simulink model "Copy_of_Ball_Estimation_27_12_new"  (Simulink 8.0)
settings: Solver=ode4  StartTime=0.0  StopTime=inf  FixedStep=sample_time  RelTol=1e-3
InitFcn:
  | sample_time=0.005;%0.004;%0.0025;%0.02;
  | sample_time_Vicon = 0.005;
  | DeltaT = 0.02;
  | g = 9.81;
  | H0 = g%0.3165;
  | 
  | Q6_mass = 0.7;
  | 
  | Q6_Omega_r = 1.6; %for horizon ref
  | Q6_Zeta_r = 0.5; %for horizon ref
  | Q6_Omega_r_h = 2;%for vertical ref
  | Q6_Zeta_r_h = 1; %for vertical ref
  | 
  | 
  | Q6_Omega = 1.5; %for horizon control
  | Q6_Zeta = 0.5; %for horizon control
  | Q6_Omega_h= 2; %for vertical control
  | Q6_Zeta_h = 0.7; %for vertical control
  | 
  | 
  | Q6_acc_max = 5;%horizontal max acc
  | Q6_acc_max_h = 3;%horizontal max acc
  | 
  | omega_circle = 72*pi/180;
  | omega_h = 0.1;%Ascending speed
  | PI = pi;
  | Circle_R = 2.5;
  | MAX_Height = -2;
libraries: simulink x2, dspadpt3 x2
settings Model: Creator=ttcl3  LastModifiedBy=NTU User
settings SolverCC: MaxConsecutiveMinStep=auto
settings DataIOCC: SignalLoggingSaveFormat=ModelDataLogs
settings DebuggingCC: MultiTaskRateTransMsg=warning  FcnCallInpInsideContextMsg=UseLocalSettings
settings SFSimCC: SimParseCustomCode=off
settings CodeAppCC: CustomSymbolStrType=$N$R$M_T  InternalIdentifier=Shortened
settings GRTTargetCC: CombineOutputUpdateFcns=off  GRTInterface=on

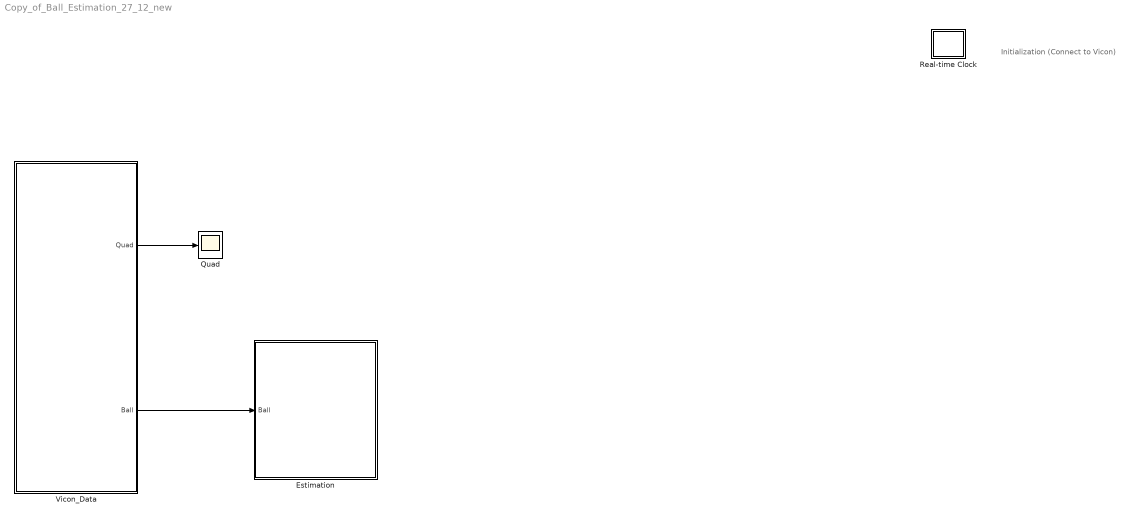
== system Copy_of_Ball_Estimation_27_12_new ==
  note: Initialization
      | (Connect to Vicon)
  Estimation : Subsystem
  Quad : Scope
      settings: YMin=0  YMax=3.25  MaxDataPoints=50000
  Real-time Clock : Subsystem  mask(Real-time Clock){sample_time=0.02, tolerance=1}
      mask prompts: sample_time "Synchronize with real-time every n seconds:"; tolerance "Real-time warning tolerance (seconds):"
      mask help: Real-time Synchronization Block
      mask Help: This block synchronizes simulation time with the PC real-time clock or UNIX system clock. The first dialog entry is the period at which the clock is checked to insure real-time synchronization. The second dialog entry is the number of seconds that the simulation time must be within real-time before a warning is printed.
      mask Display: plot(0,0,100,100,[40,60,60,54,54,64,69,76,82,77,81,83,83,81,78,74,70,64,57,49,41,35,32,30,30,31,34,40,47,47,40,40],[90,90,85,85,80,79,76,87,80,70,64,57,49,41,33,28,24,22,21,23,25,31,37,46,56,65,73,78,80,85,85,90],[69,53,53],[64,50,73])
  Vicon_Data : Subsystem
  wires:
  Vicon_Data/2(Ball) -> Estimation/1(Ball)
  Vicon_Data/1(Quad) -> Quad/1

== system Copy_of_Ball_Estimation_27_12_new/Estimation ==
  Ball : Inport
  Bus Selector1 : BusSelector  OutputSignals=Position,Velocity
  Trajectory Logic1 : Subsystem
  wires:
  Ball/1 -> Bus Selector1/1
  Bus Selector1/1 -> Trajectory Logic1/1(Ball_Pos)  "<Position>"
  Bus Selector1/2 -> Trajectory Logic1/2(Ball_Vel)  "<Velocity>"

== system Copy_of_Ball_Estimation_27_12_new/Real-time Clock ==
  Real-time Clock : S-Function  FunctionName=rtclock  Parameters=sample_time, tolerance  EnableBusSupport=off

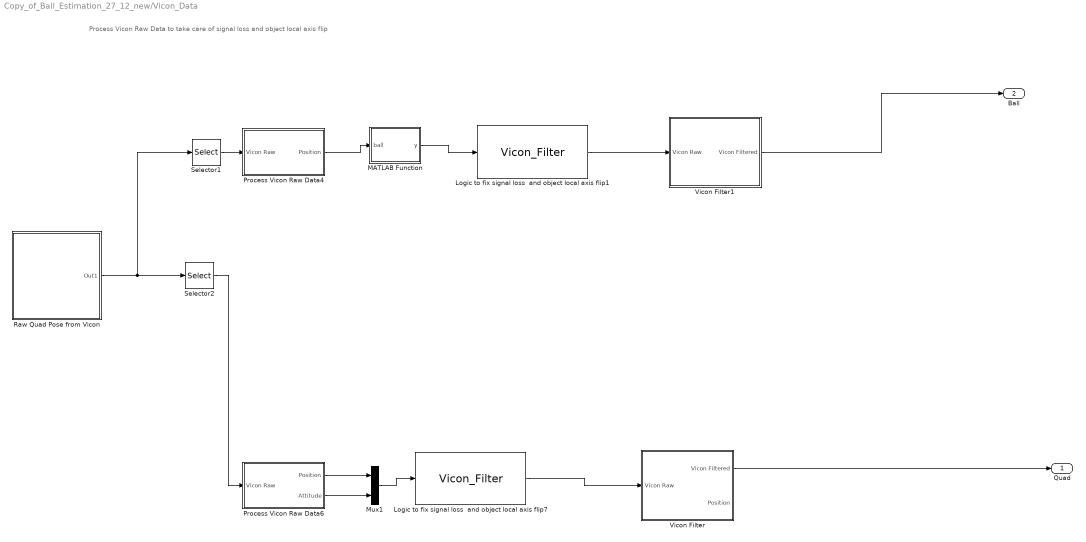
== system Copy_of_Ball_Estimation_27_12_new/Vicon_Data ==
  note: Process Vicon Raw Data to take care of signal loss and object local axis flip
  Logic to fix signal loss  and object local axis flip1 : M-S-Function  FunctionName=Vicon_Filter
  Logic to fix signal loss  and object local axis flip7 : M-S-Function  FunctionName=Vicon_Filter
  MATLAB Function : MATLAB Function  TreatAsAtomicUnit=on
  Mux1 : Mux  Inputs=2
  Process Vicon Raw Data4 : Subsystem
  Process Vicon Raw Data6 : Subsystem
  Raw Quad Pose from Vicon : Subsystem
  Selector1 : Selector  InputPortWidth=9  IndexOptions=Index vector (dialog)  Indices=[7 8 9]  OutputSizes=1
  Selector2 : Selector  InputPortWidth=9  IndexOptions=Index vector (dialog)  Indices=[1 2 3 4 5 6]  OutputSizes=1
  Vicon Filter : Subsystem  AncestorBlock=X330_Control/Vicon Filter
  Vicon Filter1 : Subsystem  AncestorBlock=X330_Control/Vicon Filter
  Quad : Outport
  Ball : Outport  Port=2
  wires:
  Selector2/1 -> Process Vicon Raw Data6/1(Vicon Raw)
  Logic to fix signal loss  and object local axis flip7/1 -> Vicon Filter/1(Vicon Raw)
  Process Vicon Raw Data6/1(Position) -> Mux1/1
  Process Vicon Raw Data6/2(Attitude) -> Mux1/2
  Mux1/1 -> Logic to fix signal loss  and object local axis flip7/1
  Vicon Filter/1(Vicon Filtered) -> Quad/1
  Process Vicon Raw Data4/1(Position) -> MATLAB Function/1(ball)
  Vicon Filter1/1(Vicon Filtered) -> Ball/1
  Raw Quad Pose from Vicon/1(Out1) -> Selector1/1, Selector2/1
  Selector1/1 -> Process Vicon Raw Data4/1(Vicon Raw)
  MATLAB Function/1(y) -> Logic to fix signal loss  and object local axis flip1/1
  Logic to fix signal loss  and object local axis flip1/1 -> Vicon Filter1/1(Vicon Raw)

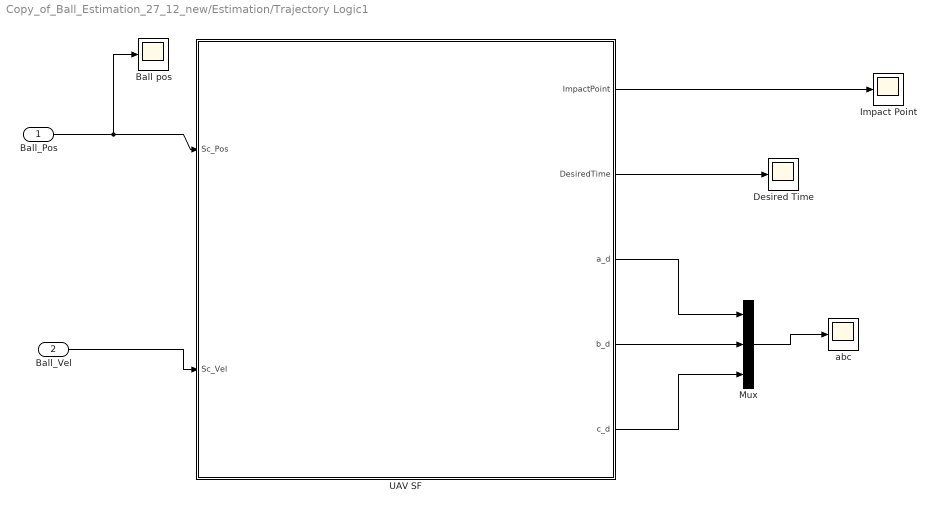
== system Copy_of_Ball_Estimation_27_12_new/Estimation/Trajectory Logic1 ==
  Ball_Pos : Inport
  Ball_Vel : Inport  Port=2
  Ball pos : Scope
      settings: TimeRange=10  YMin=-4.5  SaveName=ScopeData4  MaxDataPoints=50000
  Desired Time : Scope
      settings: TimeRange=14.55830388692581  YMin=-0.05018891687657431  YMax=0.1552267002518891  SaveName=ScopeData5  MaxDataPoints=50000
  Impact Point : Scope
      settings: TimeRange=1.719691973284533  YMin=-3.5  YMax=3.5  SaveName=ScopeData2  MaxDataPoints=50000
  Mux : Mux  Inputs=3
  UAV SF : Stateflow chart  TreatAsAtomicUnit=on
  abc : Scope
      settings: YMin=-0.25  YMax=4.5  MaxDataPoints=50000
  wires:
  Ball_Pos/1 -> Ball pos/1, UAV SF/1(Sc_Pos)
  Ball_Vel/1 -> UAV SF/2(Sc_Vel)
  UAV SF/2(DesiredTime) -> Desired Time/1
  UAV SF/3(a_d) -> Mux/1
  UAV SF/4(b_d) -> Mux/2
  UAV SF/5(c_d) -> Mux/3
  Mux/1 -> abc/1
  UAV SF/1(ImpactPoint) -> Impact Point/1

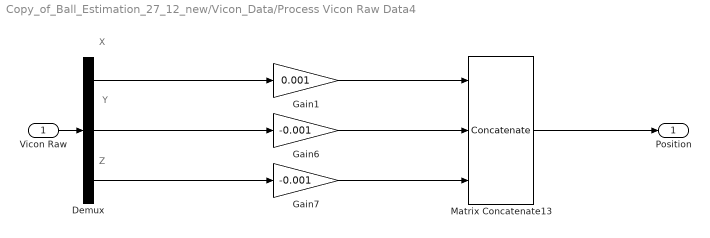
== system Copy_of_Ball_Estimation_27_12_new/Vicon_Data/Process Vicon Raw Data4 ==
  note: X
  note: Y
  note: Z
  Vicon Raw : Inport
  Demux : Demux  Outputs=3
  Gain1 : Gain  Gain=0.001
  Gain6 : Gain  Gain=-0.001
  Gain7 : Gain  Gain=-0.001
  Matrix Concatenate13 : Concatenate  NumInputs=3  Mode=Multidimensional array
  Position : Outport
  wires:
  Gain1/1 -> Matrix Concatenate13/1
  Demux/1 -> Gain1/1
  Demux/2 -> Gain6/1
  Demux/3 -> Gain7/1
  Gain6/1 -> Matrix Concatenate13/2
  Gain7/1 -> Matrix Concatenate13/3
  Matrix Concatenate13/1 -> Position/1
  Vicon Raw/1 -> Demux/1

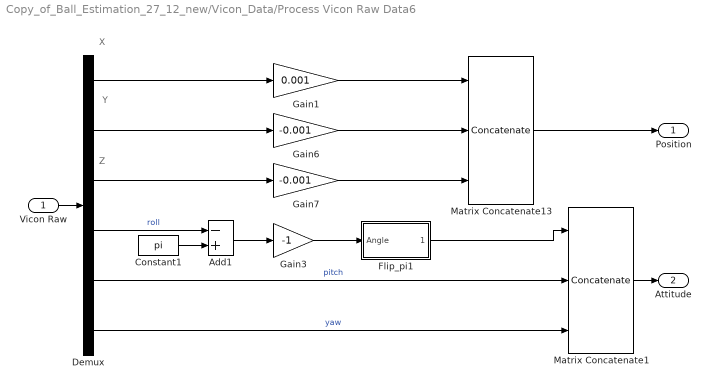
== system Copy_of_Ball_Estimation_27_12_new/Vicon_Data/Process Vicon Raw Data6 ==
  note: X
  note: Y
  note: Z
  Vicon Raw : Inport
  Add1 : Sum  Inputs=-+
  Constant1 : Constant  Value=pi  OutDataTypeStr=double
  Demux : Demux  Outputs=6
  Flip_pi1 : Subsystem  mask(Flip -pi to pi){}
      mask help: Flips the inputs into the range -pi to pi
      mask Help: Flips the inputs into the range -pi to pi
      mask Display: disp('Flip_pi')
  Gain1 : Gain  Gain=0.001
  Gain3 : Gain  Gain=-1
  Gain6 : Gain  Gain=-0.001
  Gain7 : Gain  Gain=-0.001
  Matrix Concatenate1 : Concatenate  NumInputs=3  Mode=Multidimensional array
  Matrix Concatenate13 : Concatenate  NumInputs=3  Mode=Multidimensional array
  Position : Outport
  Attitude : Outport  Port=2
  wires:
  Constant1/1 -> Add1/2
  Demux/6 -> Matrix Concatenate1/3  "yaw"
  Gain1/1 -> Matrix Concatenate13/1
  Demux/1 -> Gain1/1
  Demux/2 -> Gain6/1
  Demux/3 -> Gain7/1
  Demux/4 -> Add1/1  "roll"
  Gain6/1 -> Matrix Concatenate13/2
  Gain7/1 -> Matrix Concatenate13/3
  Add1/1 -> Gain3/1
  Gain3/1 -> Flip_pi1/1(Angle)
  Demux/5 -> Matrix Concatenate1/2  "pitch"
  Flip_pi1/1(Angle_Flip) -> Matrix Concatenate1/1
  Matrix Concatenate13/1 -> Position/1
  Vicon Raw/1 -> Demux/1
  Matrix Concatenate1/1 -> Attitude/1

== system Copy_of_Ball_Estimation_27_12_new/Vicon_Data/Raw Quad Pose from Vicon ==
  Constant : Constant
  Interpreted MATLAB Function : MATLABFcn  MATLABFcn=GetViconPose_BallCatching_mae_lab  OutputDimensions=9  SampleTime=0.005
  Out1 : Outport
  wires:
  Constant/1 -> Interpreted MATLAB Function/1
  Interpreted MATLAB Function/1 -> Out1/1

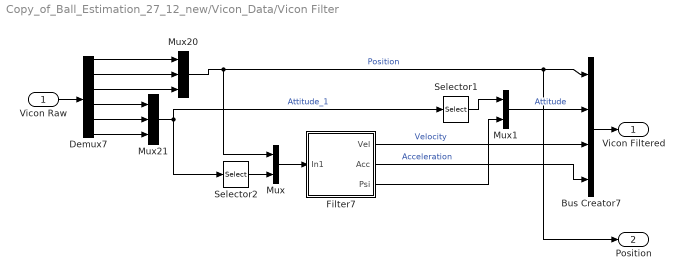
== system Copy_of_Ball_Estimation_27_12_new/Vicon_Data/Vicon Filter ==
  Vicon Raw : Inport
  Bus Creator7 : BusCreator
  Demux7 : Demux  Outputs=6
  Filter7 : Subsystem
  Mux : Mux  Inputs=2
  Mux1 : Mux  Inputs=2
  Mux20 : Mux  Inputs=3
  Mux21 : Mux  Inputs=3
  Selector1 : Selector  InputPortWidth=3  IndexOptions=Index vector (dialog)  Indices=[1 2]  OutputSizes=1
  Selector2 : Selector  InputPortWidth=3  IndexOptions=Index vector (dialog)  Indices=[3]  OutputSizes=1
  Vicon Filtered : Outport
  Position : Outport  Port=2
  wires:
  Bus Creator7/1 -> Vicon Filtered/1
  Vicon Raw/1 -> Demux7/1
  Mux1/1 -> Bus Creator7/2  "Attitude"
  Selector1/1 -> Mux1/1
  Filter7/3(Psi) -> Mux1/2
  Mux/1 -> Filter7/1(In1)
  Selector2/1 -> Mux/2
  Filter7/2(Acc) -> Bus Creator7/4  "Acceleration"
  Filter7/1(Vel) -> Bus Creator7/3  "Velocity"
  Mux21/1 -> Selector1/1, Selector2/1  "Attitude_1"
  Mux20/1 -> Mux/1, Position/1, Bus Creator7/1  "Position"
  Demux7/2 -> Mux20/2
  Demux7/1 -> Mux20/1
  Demux7/6 -> Mux21/3
  Demux7/5 -> Mux21/2
  Demux7/4 -> Mux21/1
  Demux7/3 -> Mux20/3

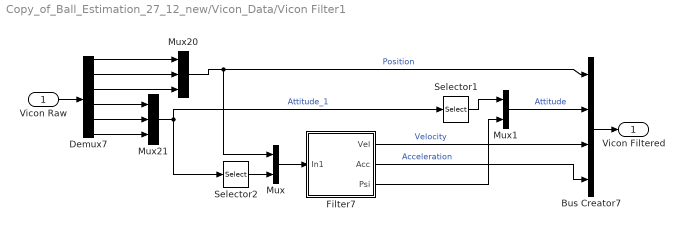
== system Copy_of_Ball_Estimation_27_12_new/Vicon_Data/Vicon Filter1 ==
  Vicon Raw : Inport
  Bus Creator7 : BusCreator
  Demux7 : Demux  Outputs=6
  Filter7 : Subsystem
  Mux : Mux  Inputs=2
  Mux1 : Mux  Inputs=2
  Mux20 : Mux  Inputs=3
  Mux21 : Mux  Inputs=3
  Selector1 : Selector  InputPortWidth=3  IndexOptions=Index vector (dialog)  Indices=[1 2]  OutputSizes=1
  Selector2 : Selector  InputPortWidth=3  IndexOptions=Index vector (dialog)  Indices=[3]  OutputSizes=1
  Vicon Filtered : Outport
  wires:
  Demux7/3 -> Mux20/3
  Demux7/4 -> Mux21/1
  Demux7/5 -> Mux21/2
  Demux7/6 -> Mux21/3
  Demux7/1 -> Mux20/1
  Demux7/2 -> Mux20/2
  Mux20/1 -> Bus Creator7/1, Mux/1  "Position"
  Mux21/1 -> Selector2/1, Selector1/1  "Attitude_1"
  Filter7/1(Vel) -> Bus Creator7/3  "Velocity"
  Filter7/2(Acc) -> Bus Creator7/4  "Acceleration"
  Selector2/1 -> Mux/2
  Mux/1 -> Filter7/1(In1)
  Filter7/3(Psi) -> Mux1/2
  Selector1/1 -> Mux1/1
  Mux1/1 -> Bus Creator7/2  "Attitude"
  Vicon Raw/1 -> Demux7/1
  Bus Creator7/1 -> Vicon Filtered/1

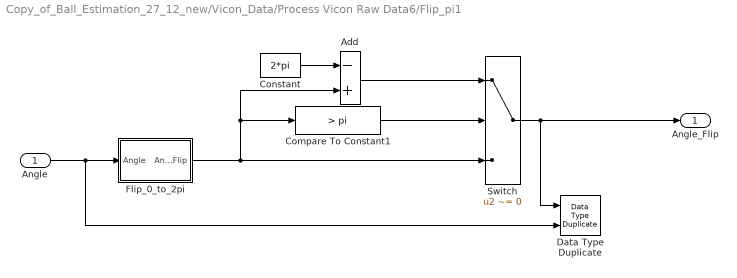
== system Copy_of_Ball_Estimation_27_12_new/Vicon_Data/Process Vicon Raw Data6/Flip_pi1 ==
  Angle : Inport
  Add : Sum  Inputs=-+
  Compare To Constant1 : simulink/Logic and Bit Operations/Compare To Constant  relop=>  const=pi  OutDataTypeStr=uint8  ZeroCross=off
  Constant : Constant  Value=2*pi
  Data Type Duplicate : DataTypeDuplicate
  Flip_0_to_2pi : Subsystem  mask(Flip zero to 2pi){}
      mask help: Flips the inputs into the range zero to +2pi
      mask Help: Flips the inputs into the range zero to +2pi
      mask Display: disp('Flip_0_2pi')
  Switch : Switch  Criteria=u2 ~= 0
  Angle_Flip : Outport
  wires:
  Switch/1 -> Data Type Duplicate/1, Angle_Flip/1
  Add/1 -> Switch/1
  Constant/1 -> Add/1
  Compare To Constant1/1 -> Switch/2
  Flip_0_to_2pi/1(Angle_Flip) -> Add/2, Compare To Constant1/1, Switch/3
  Angle/1 -> Data Type Duplicate/2, Flip_0_to_2pi/1(Angle)

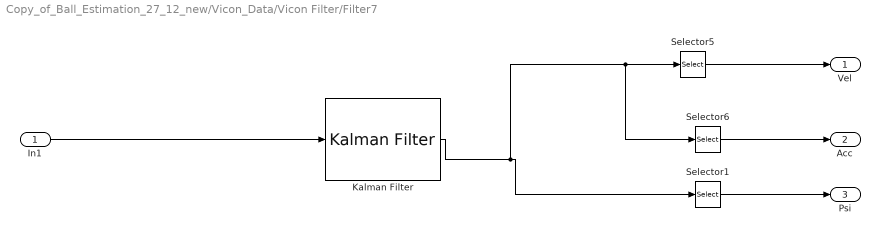
== system Copy_of_Ball_Estimation_27_12_new/Vicon_Data/Vicon Filter/Filter7 ==
  In1 : Inport
  Kalman Filter : dspadpt3/Kalman Filter  num_targets=1  sourceEnable=Always  isReset=on  X=zeros([12, 1])  P=zeros(12)  A=[1 sample_time_Vicon sample_time_Vicon*sample_time_Vicon/2 zeros(1,9);0 1 sample_time_Vicon zeros(1,9);0 0 1 zeros(1,9);0 0 0 1 sample_time_Vicon sample_time_Vicon*sample_time_Vicon/2 zeros(1,6);zeros(1,4) 1 sample_time_Vicon zeros(1,6);zeros(1,5) 1 zeros(1,6);zeros(1,6) 1 sample_time_Vicon sample_time_Vicon*sample_time_Vicon/2 zeros(1,3);zeros(1,7) 1 sample_time_Vicon zeros(1,3);zeros(1,8) 1 zeros(1,3);zeros(1,9) 1 sample_time_Vicon sample_time_Vicon*sample_time_Vicon/2;zeros(1,10) 1 sample_time_Vicon;zeros(1,11) 1];  sourceMeasure=Specify via Dialog  H=[1 zeros(1,11); zeros(1,3) 1 zeros(1,8);zeros(1,6) 1 zeros(1,5);zeros(1,9) 1 0 0]  Q=diag([0 0.001 0.001 0 0.001 0.001 0 0.001 0.001 0 0.001 0.001]);  R=diag([0.001 0.001 0.001 0.05])  isOutputEstMeasure=off  isOutputEstState=on  isOutputEstError=off  isOutputPrdMeasure=off  isOutputPrdState=off  isOutputPrdError=off
  Selector1 : Selector  InputPortWidth=12  IndexOptions=Index vector (dialog)  Indices=[10]  OutputSizes=1
  Selector5 : Selector  InputPortWidth=12  IndexOptions=Index vector (dialog)  Indices=[2 5 8]  OutputSizes=1
  Selector6 : Selector  InputPortWidth=12  IndexOptions=Index vector (dialog)  Indices=[3 6 9]  OutputSizes=1
  Vel : Outport
  Acc : Outport  Port=2
  Psi : Outport  Port=3
  wires:
  Selector1/1 -> Psi/1
  Selector5/1 -> Vel/1
  In1/1 -> Kalman Filter/1
  Kalman Filter/1 -> Selector1/1, Selector5/1, Selector6/1
  Selector6/1 -> Acc/1

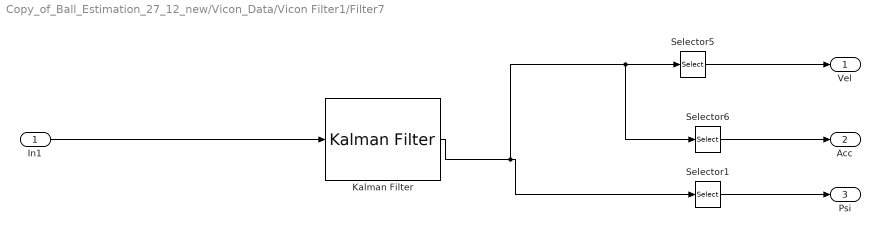
== system Copy_of_Ball_Estimation_27_12_new/Vicon_Data/Vicon Filter1/Filter7 ==
  In1 : Inport
  Kalman Filter : dspadpt3/Kalman Filter  num_targets=1  sourceEnable=Always  isReset=on  X=zeros([12, 1])  P=zeros(12)  A=[1 sample_time_Vicon sample_time_Vicon*sample_time_Vicon/2 zeros(1,9);0 1 sample_time_Vicon zeros(1,9);0 0 1 zeros(1,9);0 0 0 1 sample_time_Vicon sample_time_Vicon*sample_time_Vicon/2 zeros(1,6);zeros(1,4) 1 sample_time_Vicon zeros(1,6);zeros(1,5) 1 zeros(1,6);zeros(1,6) 1 sample_time_Vicon sample_time_Vicon*sample_time_Vicon/2 zeros(1,3);zeros(1,7) 1 sample_time_Vicon zeros(1,3);zeros(1,8) 1 zeros(1,3);zeros(1,9) 1 sample_time_Vicon sample_time_Vicon*sample_time_Vicon/2;zeros(1,10) 1 sample_time_Vicon;zeros(1,11) 1];  sourceMeasure=Specify via Dialog  H=[1 zeros(1,11); zeros(1,3) 1 zeros(1,8);zeros(1,6) 1 zeros(1,5);zeros(1,9) 1 0 0]  Q=diag([0 0.001 0.001 0 0.001 0.001 0 0.001 0.001 0 0.001 0.001]);  R=diag([0.001 0.001 0.001 0.05])  isOutputEstMeasure=off  isOutputEstState=on  isOutputEstError=off  isOutputPrdMeasure=off  isOutputPrdState=off  isOutputPrdError=off
  Selector1 : Selector  InputPortWidth=12  IndexOptions=Index vector (dialog)  Indices=[10]  OutputSizes=1
  Selector5 : Selector  InputPortWidth=12  IndexOptions=Index vector (dialog)  Indices=[2 5 8]  OutputSizes=1
  Selector6 : Selector  InputPortWidth=12  IndexOptions=Index vector (dialog)  Indices=[3 6 9]  OutputSizes=1
  Vel : Outport
  Acc : Outport  Port=2
  Psi : Outport  Port=3
  wires:
  Selector6/1 -> Acc/1
  Kalman Filter/1 -> Selector6/1, Selector5/1, Selector1/1
  In1/1 -> Kalman Filter/1
  Selector5/1 -> Vel/1
  Selector1/1 -> Psi/1

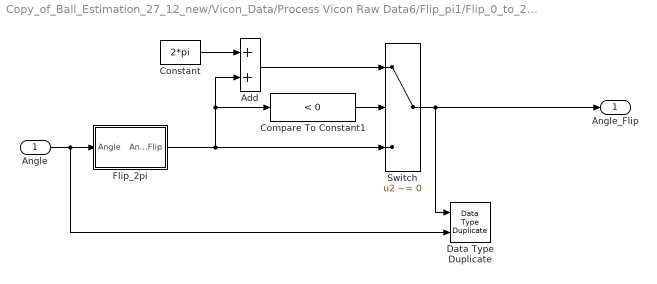
== system Copy_of_Ball_Estimation_27_12_new/Vicon_Data/Process Vicon Raw Data6/Flip_pi1/Flip_0_to_2pi ==
  Angle : Inport
  Add : Sum
  Compare To Constant1 : simulink/Logic and Bit Operations/Compare To Constant  relop=<  const=0  OutDataTypeStr=uint8  ZeroCross=off
  Constant : Constant  Value=2*pi
  Data Type Duplicate : DataTypeDuplicate
  Flip_2pi : Subsystem  mask(Flip -2pi to 2pi){}
      mask help: Flips the inputs into the range -2pi to +2pi
      mask Help: Flips the inputs into the range -2pi to +2pi
      mask Display: disp('Flip_2pi')
  Switch : Switch  Criteria=u2 ~= 0
  Angle_Flip : Outport
  wires:
  Switch/1 -> Data Type Duplicate/1, Angle_Flip/1
  Angle/1 -> Data Type Duplicate/2, Flip_2pi/1(Angle)
  Add/1 -> Switch/1
  Constant/1 -> Add/1
  Compare To Constant1/1 -> Switch/2
  Flip_2pi/1(Angle_Flip) -> Switch/3, Add/2, Compare To Constant1/1

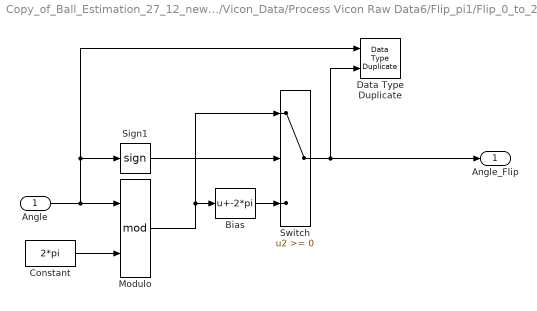
== system Copy_of_Ball_Estimation_27_12_new/Vicon_Data/Process Vicon Raw Data6/Flip_pi1/Flip_0_to_2pi/Flip_2pi ==
  Angle : Inport
  Bias : Bias  Bias=-2*pi
  Constant : Constant  Value=2*pi
  Data Type Duplicate : DataTypeDuplicate
  Modulo : Math  Operator=mod  SaturateOnIntegerOverflow=on
  Sign1 : Signum
  Switch : Switch
  Angle_Flip : Outport
  wires:
  Switch/1 -> Data Type Duplicate/2, Angle_Flip/1
  Bias/1 -> Switch/3
  Sign1/1 -> Switch/2
  Modulo/1 -> Switch/1, Bias/1
  Constant/1 -> Modulo/2
  Angle/1 -> Data Type Duplicate/1, Sign1/1, Modulo/1

== matlab function Vicon_Data/MATLAB Function ==
  data: ball input double; y output double
function y = fcn(ball)
%#codegen
temp = zeros(3,1);

for i=1:3;
   temp(i) = ball(i);     
end;
y = zeros(6,1);
y(1) = temp(1);
y(2) = temp(2);
y(3) = temp(3);
y(4) = 0;
y(5) = 0;
y(6) = 0;
end

== stateflow chart Estimation/Trajectory Logic1/UAV SF ==
  state Airborne
    state Standby
    state Calculation
      en:
      [Pe,T,a_1,b_1,c]=TrajEst(x,y,z,zd,Peo[0],Peo[1],To);
      x[0] = x[1];x[1] = x[2];x[2] = x[3];x[3] = x[4];
      y[0] = y[1];y[1] = y[2];y[2] = y[3];y[3] = y[4];
      z[0] = z[1];z[1] = z[2];z[2] = z[3];z[3] = z[4];
    state Getdata
      en:
      x[i] = Sc_Pos[0];
      y[i] = Sc_Pos[1];
      z[i] = Sc_Pos[2];
    state Output1
      en:
      ImpactPoint = Pe;
      DesiredTime = T;
      a_d=a_1;
      b_d=b_1;
      c_d=c;
    state daq
      en:
      i=i+1;
    state Output2
      en:
      ImpactPoint[0] = 0;
      ImpactPoint[1] = 0;
      ImpactPoint[2] = zd;
      DesiredTime = 0;
    Output1 -> (junction 18) : {i=i-2;}
    (default) -> Standby : {i=-1;Peo=0;To=0;}
    (junction 19) -> (junction 18) [order 1] : [(Sc_Vel[2]<-0.5)&(Sc_Vel[2]>-6)]
    Standby -> (junction 19) : [(abs(Sc_Pos[0]) <= 4.5)&(abs(Sc_Pos[1])<=4.5)&(abs(Sc_Pos[2])<=4)]
    (junction 18) -> daq [order 2]
    (junction 19) -> Output2 [order 2]
    Output2 -> Standby
    (junction 18) -> Output2 [order 1] : [(Sc_Pos[2] >= -0.8)&(Sc_Vel[2]>0)]
    Getdata -> daq
    daq -> Getdata [order 1] : [i==0]
    (junction 20) -> Getdata [order 1] : [(x[i-1]~=Sc_Pos[0])||(y[i-1]~=Sc_Pos[1])||(z[i-1]~=Sc_Pos[2])]
    daq -> (junction 20) [order 3] : [(i>0)&(i<5)]
    (junction 20) -> daq [order 2] : {i=i-1;}
    daq -> Calculation [order 2] : [i==5]
    Calculation -> Output1 : {Peo=Pe;To=T;}
  data: xi function_input double size=5; yi function_input double size=5; zi function_input double size=5; Pe function_output double size=3; T function_output double size=1; zd function_input double size=1; t0 constant double size=5 =[0 0.005 0.01 0.015 0.02]; xo function_input double; yo function_input double; To function_input double; a_1 function_output double size=1; b_1 function_output double size=1; c function_output double size=1; ImpactPoint output double size=3; DesiredTime output double size=1; Sc_Pos input double size=3; Sc_Vel input double size=3; DeltaT parameter double size=1; T local double size=1; zd local double size=1 =-0.8; Pe local double size=3; i local double; x local double size=5 =[0 0 0 0 0 ]; y local double size=5 =[0 0 0 0 0 ]; z local double size=5 =[0 0 0 0 0 ]; Peo local double size=3; To local double size=1; Pe1 local double size=3; T1 local double size=1; a_d output double size=1; b_d output double size=1; c_d output double size=1; a_1 local double; b_1 local double; c local double
  function [Pe,T,a_1,b_1,c] =TrajEst(xi,yi,zi,zd,xo,yo,To):
    | function [Pe,T,a_1,b_1,c] =TrajEst(xi,yi,zi,zd,xo,yo,To)
    | 
    | p=polyfit(t0,zi,2)';
    | a=p(1);
    | b=p(2);
    | c=p(3);
    | 
    | r=polyfit(t0,xi,1)';
    | a_1=r(1);
    | b_1=r(2);
    | 
    | xe=0;
    | ye=0;
    | T=0;
    | if((To>0)&&(To<1.2))
    |     xe = xo;
    |     ye = yo;
    |     T = To;
    | end;
    | if(a > 3)
    |     if(b^2 - 4*a*(c-zd) >= 0)
    |         T=(-b+sqrt(b^2 - 4*a*(c-zd)))/(2*a);
    |                 xe=polyval(polyfit(t0,xi,1),0.9*T);
    |         ye=polyval(polyfit(t0,yi,1),0.9*T);
    |     end;
    | 
    |     if((To>0)&&(To<1.2))
    |         if((T>1.2)||(abs(xe)>4)||(abs(ye)>4))
    |             T = To;
    |             xe = xo;
    |             ye = yo;
    |         else
    |             T = 0.7*T + 0.3*(To-0.005);
    |             xe = 0.3*xo + 0.7*xe;
    |             ye = 0.3*yo + 0.7*ye;
    |         end
    |     else
    |        if((T>1.2)||(xe<-1.5)||(xe>2.5)||(ye<-2.5)||(ye>2.5)) 
    |            xe=0;
    |            ye=0;
    |            T=0;
    |        end;
    |     end;
    | end
    | 
    | Pe=[xe ye zd]';
